simulink library "mech_conveyor_vrlib"  (Simulink 7.1)
libraries: mblibv1 x4, vrlib x1
settings Model: Creator=arnav  LastModifiedBy=batserve

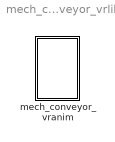
== system mech_conveyor_vrlib ==
  mech_conveyor_vranim : Subsystem

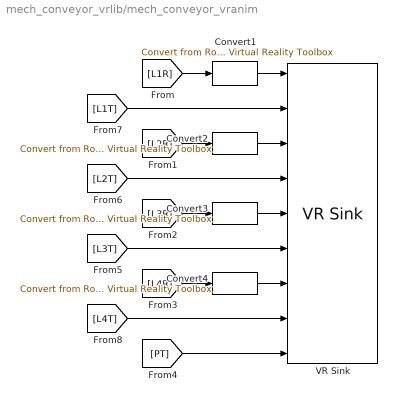
== system mech_conveyor_vrlib/mech_conveyor_vranim ==
  Convert{1..4} (4 alike) : mblibv1/Utilities/Convert from Rotation Matrix to Virtual Reality Toolbox  Tag=Pose2VR
  VR Sink : vrlib/VR Sink  SampleTime=0.1  ViewEnable=on  RemoteChange=off  RemoteView=off  FieldsWritten=Link1.rotation.4#Link1.translation.3#Link2.rotation.4#Link2.translation.3#Link3.rotation.4#Link3.translation.3#Link4.rotation.4#Link4.translation.3#Pusher.translation.3  WorldFileName=convmech.wrl  WorldDescription=convmech  AutoView=off  FigureProperties={}
  wires:
  [PT] -> VR Sink/9
  [L4T] -> VR Sink/8
  Convert1/1 -> VR Sink/1
  Convert4/1 -> VR Sink/7
  [L3T] -> VR Sink/6
  Convert3/1 -> VR Sink/5
  [L2T] -> VR Sink/4
  Convert2/1 -> VR Sink/3
  [L1T] -> VR Sink/2
  [L4R] -> Convert4/1
  [L3R] -> Convert3/1
  [L2R] -> Convert2/1
  [L1R] -> Convert1/1
